simulink model "RTP_V1_Corona_Temperaturregelung_Simu_V7_Vorlage"  (R2018b)
settings: Solver=VariableStepAuto  StartTime=0.0  StopTime=500  FixedStep=0.01  RelTol=1e-3  EnableMultiTasking=on
values from neighbouring files (symbols this model uses):
  K_P = 0.5*K_krit    [RTP_V1_Corona_Belege_Variablen_Regler_V7_Vorlage.m]
undefined symbols (not defined in the file or in its folder): sigbuilder_block
settings Model: Creator=gregor  LastModifiedBy=gregor
settings DataIOCC: LimitDataPoints=on  SaveFormat=Array  SignalLoggingSaveFormat=ModelDataLogs  SaveState=on
settings OptimizationCC: ExpressionDepthLimit=2147483647  InitFltsAndDblsToZero=on  LifeSpan=inf
settings DebuggingCC: SaveWithParameterizedLinksMsg=none  UnderspecifiedInitializationDetection=Classic  MergeDetectMultiDrivingBlocksExec=none  SignalResolutionControl=TryResolveAllWithWarning  SolverPrmCheckMsg=warning  MultiTaskDSMMsg=warning  MultiTaskCondExecSysMsg=none  FcnCallInpInsideContextMsg=warning  ModelReferenceExtraNoncontSigs=none  StateNameClashWarn=warning  LibraryContextMissingDiagnostic=none  SFUnexpectedBacktrackingDiag=warning  SFNoUnconditionalDefaultTransitionDiag=warning  SFExecutionAtInitializationDiag=none
settings HardwareCC: ProdBitPerPointer=32  ProdBitPerSizeT=32  ProdBitPerPtrDiffT=32  ProdLargestAtomicFloat=None  ProdIntDivRoundTo=Undefined  ProdEndianess=Unspecified  ProdWordSize=32  ProdHWDeviceType=32-bit Generic
settings ModelReferenceCC: PropagateSignalLabelsOutOfModel=off
settings SFSimCC: SimUseLocalCustomCode=off
settings RTWCC: RTWUseLocalCustomCode=off
settings CodeAppCC: StateflowObjectComments=on
settings GRTTargetCC: TargetFcnLib=ansi_tfl_tmw.mat  TargetLangStandard=C89/C90 (ANSI)  GeneratePreprocessorConditionals=Disable all  CombineOutputUpdateFcns=off  GRTInterface=on
settings ConfigComp: CovMetricSettings=dw  CovHtmlReporting=on  CovSaveCumulativeToWorkspaceVar=on  CovSaveSingleToWorkspaceVar=on  CovExternalEMLEnable=off

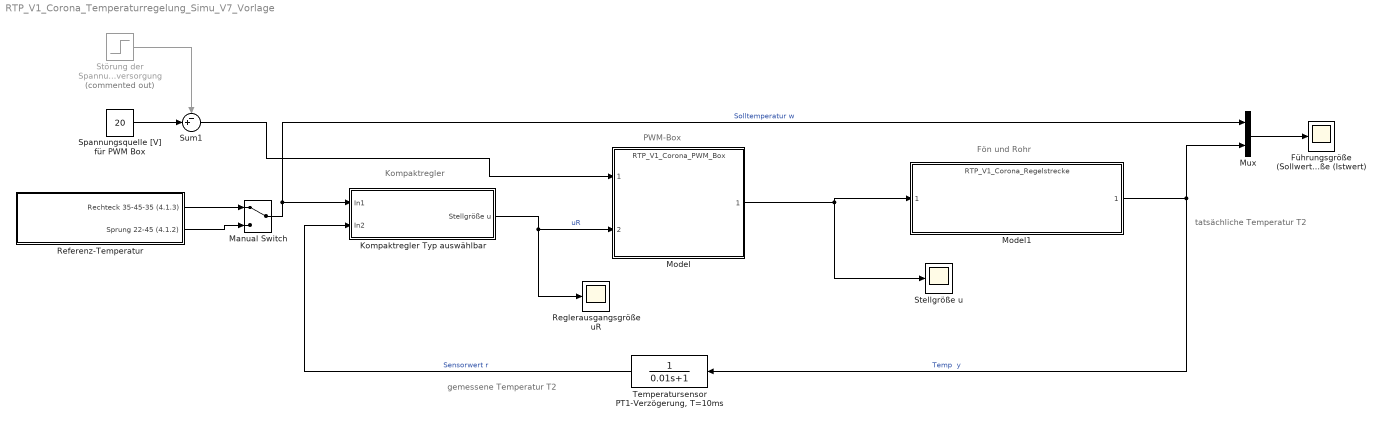
== system RTP_V1_Corona_Temperaturregelung_Simu_V7_Vorlage ==
  note: Fön und Rohr
  note: PWM-Box
  note: tatsächliche
      | Temperatur T2
  note: gemessene
      | Temperatur T2
  note: Kompaktregler
  "Führungsgröße (Sollwert) Regelgröße (Istwert) " : Scope
  "Kompaktregler Typ auswählbar " : Subsystem  mask{K=K_P, Tn=1, I_aktiv=off, Tv=1, D_aktiv=off}
      mask prompts: K "Verstärkung (K)"; Tn "Nachlaufzeit (T_n)"; I_aktiv "I-Anteil aktivieren"; Tv "Vorhaltzeit (T_v)"; D_aktiv "D-Anteil aktivieren"
      mask help:
      | PID-Regler:
      |
      | G_R(s) = K(1 + 1/(s*T_n) + T_v*s)
      mask Help:
      | PID-Regler:
      | 
      | G_R(s) = K(1 + 1/(s*T_n) + T_v*s)
  Manual Switch : ManualSwitch
  Model : ModelReference  ModelNameDialog=RTP_V1_Corona_PWM_Box.slxp  ModelReferenceVersion=1.152  CopyOfModelProtected=on
  Model1 : ModelReference  ModelNameDialog=RTP_V1_Corona_Regelstrecke.slxp  ModelReferenceVersion=1.152  CopyOfModelProtected=on
  Mux : Mux  Inputs=2
  Referenz-Temperatur : Subsystem  Tag=STV Subsys  LoadFcn=sigbuilder_block('load');  StartFcn=sigbuilder_block('start');  StopFcn=sigbuilder_block('stop');  ClipboardFcn=sigbuilder_block('clipboard');  mask(Sigbuilder block){tuvar=[0:10]}
      mask help: Simulink:masks:SigbuilderBlock_MD
      mask init:
      | if ~strcmp(get_param(bdroot(gcbh),'SimulationStatus'),'stopped') tuvar = sigbuilder_block('maskInit'); end
      settings: CopyFcn=sigbuilder_block('copy');  DeleteFcn=sigbuilder_block('delete');  ModelCloseFcn=sigbuilder_block('modelClose');  PreSaveFcn=sigbuilder_block('preSave');  PauseFcn=sigbuilder_block('pause');  ContinueFcn=sigbuilder_block('continue');  NameChangeFcn=sigbuilder_block('namechange');  OpenFcn=sigbuilder_block('open',[152.25 106.5 550.5 505.5 ]);  CloseFcn=sigbuilder_block('close');
      mask Display: plot(0, 0, 100, 100,[2, 2, 32, 32, 2], [68, 8, 8, 68, 68],[32, 2], [38, 38], [32, 19, 2],[53, 60, 44], [32, 17, 17, 2],[16, 16, 31, 31]);txt = getActiveGroup(gcbh);text(2, 100, txt,'verticalAlignment', 'top');
  Reglerausgangsgröße uR : Scope
  Spannungsquelle [V] für PWM Box : Constant  Value=20
  Stellgröße u : Scope
  Störung der Spannungsversorgung : Step  Commented=on  Time=250  After=3  SampleTime=0
  Sum1 : Sum  Inputs=-+|
  "Temperatursensor PT1-Verzögerung, T=10ms" : TransferFcn  Denominator=[0.01 1]
  wires:
  Mux/1 -> "Führungsgröße (Sollwert) Regelgröße (Istwert) "/1
  Model1/1 -> "Temperatursensor PT1-Verzögerung, T=10ms"/1, Mux/2  "Temp  y"
  Spannungsquelle [V] für PWM Box/1 -> Sum1/2
  Störung der Spannungsversorgung/1 -> Sum1/1
  "Kompaktregler Typ auswählbar "/1(Stellgröße u) -> Reglerausgangsgröße uR/1, Model/2  "uR"
  Referenz-Temperatur/2(Sprung 22-45 (4.1.2)) -> Manual Switch/2
  Referenz-Temperatur/1(Rechteck 35-45-35 (4.1.3)) -> Manual Switch/1
  Manual Switch/1 -> "Kompaktregler Typ auswählbar "/1(In1), Mux/1  "Solltemperatur w"
  Model/1 -> Stellgröße u/1, Model1/1
  "Temperatursensor PT1-Verzögerung, T=10ms"/1 -> "Kompaktregler Typ auswählbar "/2(In2)  "Sensorwert r"
  Sum1/1 -> Model/1

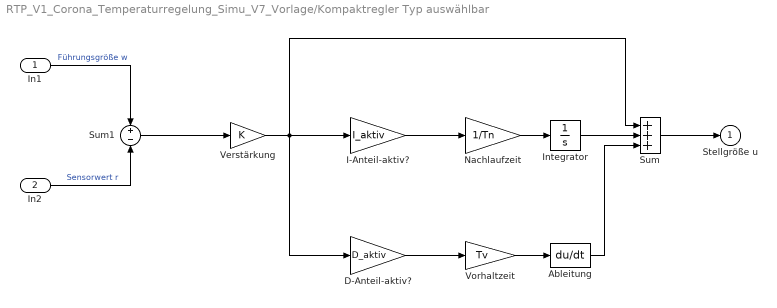
== system RTP_V1_Corona_Temperaturregelung_Simu_V7_Vorlage/Kompaktregler Typ auswählbar  ==
  In1 : Inport
  In2 : Inport  Port=2
  Ableitung : Derivative  CoefficientInTFapproximation=0.01
  "D-Anteil-aktiv? " : Gain  Gain=D_aktiv  SaturateOnIntegerOverflow=on  OutDataTypeStr=Inherit: Same as input  ParamDataTypeStr=Inherit: Same as input
  "I-Anteil-aktiv? " : Gain  Gain=I_aktiv  SaturateOnIntegerOverflow=on  OutDataTypeStr=Inherit: Same as input  ParamDataTypeStr=Inherit: Same as input
  Integrator : Integrator  LimitOutput=on  UpperSaturationLimit=1  LowerSaturationLimit=-1
  Nachlaufzeit : Gain  Gain=1/Tn  SaturateOnIntegerOverflow=on  OutDataTypeStr=Inherit: Same as input  ParamDataTypeStr=Inherit: Same as input
  Sum : Sum  Inputs=+++  SaturateOnIntegerOverflow=on  InputSameDT=on  OutDataTypeStr=Inherit: Same as first input
  Sum1 : Sum  Inputs=+|-
  Verstärkung : Gain  Gain=K  SaturateOnIntegerOverflow=on  OutDataTypeStr=Inherit: Same as input  ParamDataTypeStr=Inherit: Same as input
  Vorhaltzeit : Gain  Gain=Tv  SaturateOnIntegerOverflow=on  OutDataTypeStr=Inherit: Same as input  ParamDataTypeStr=Inherit: Same as input
  Stellgröße u : Outport  InitialOutput=0
  wires:
  Integrator/1 -> Sum/2
  Ableitung/1 -> Sum/3
  Sum/1 -> Stellgröße u/1
  Vorhaltzeit/1 -> Ableitung/1
  Sum1/1 -> Verstärkung/1
  Verstärkung/1 -> "D-Anteil-aktiv? "/1, "I-Anteil-aktiv? "/1, Sum/1
  Nachlaufzeit/1 -> Integrator/1
  "I-Anteil-aktiv? "/1 -> Nachlaufzeit/1
  "D-Anteil-aktiv? "/1 -> Vorhaltzeit/1
  In1/1 -> Sum1/1  "Führungsgröße w"
  In2/1 -> Sum1/2  "Sensorwert r"

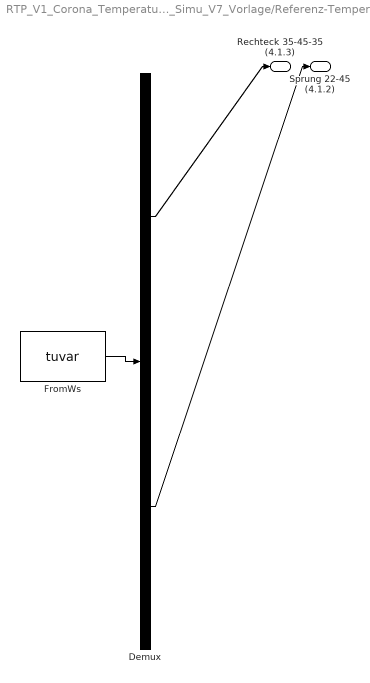
== system RTP_V1_Corona_Temperaturregelung_Simu_V7_Vorlage/Referenz-Temperatur ==
  Demux : Demux  Tag=STV Demux  Outputs=2
  FromWs : FromWorkspace  Tag=STV FromWs  VariableName=tuvar  SampleTime=0
      SigBuilderData=|
      | common.afterFinalStr = 'Extrapolate'
      | common.sampleTime = 0
      | dataSet.timeRange = [0 400]
      | dataSet.name = 'Führungsgröße'
      | sbobj.Groups.Name = 'Führungsgröße'
      | sbobj.Groups.Signals(1).Name = 'Rechteck 35-45-35 (4.1.3)'
      | sbobj.Groups.Signals(1).XData = [0 1 100 100 299.99 300 400]
      | sbobj.Groups.Signals(1).YData = [35 35 35 45 45 35 35]
      | sbobj.Groups.Signals(2).Name = 'Sprung 22-45 (4.1.2)'
      | sbobj.Groups.Signals(2).XData = [0 10 10 400]
      | sbobj.Groups.Signals(2).YData = [22 22 45 45]
      | sbobj.Groups.TimeRange = [0 400]
  Rechteck 35-45-35 (4.1.3) : Outport  Tag=STV Outport
  Sprung 22-45 (4.1.2) : Outport  Tag=STV Outport  Port=2
  wires:
  FromWs/1 -> Demux/1
  Demux/1 -> Rechteck 35-45-35 (4.1.3)/1
  Demux/2 -> Sprung 22-45 (4.1.2)/1
